simulink model "Model_2"  (R2020b)
settings: Solver=VariableStepAuto  StartTime=0.0  StopTime=10  RelTol=1e-3
values from neighbouring files (symbols this model uses):
  b1 = 350    [Variables.m]
  k1 = 80000    [Variables.m]
  k2 = 500000    [Variables.m]
  M1 = 2500    [Variables.m]
  M2 = 250    [Variables.m]
settings Model: SimulationMode=accelerator  Creator=samar  LastModifiedBy=samar

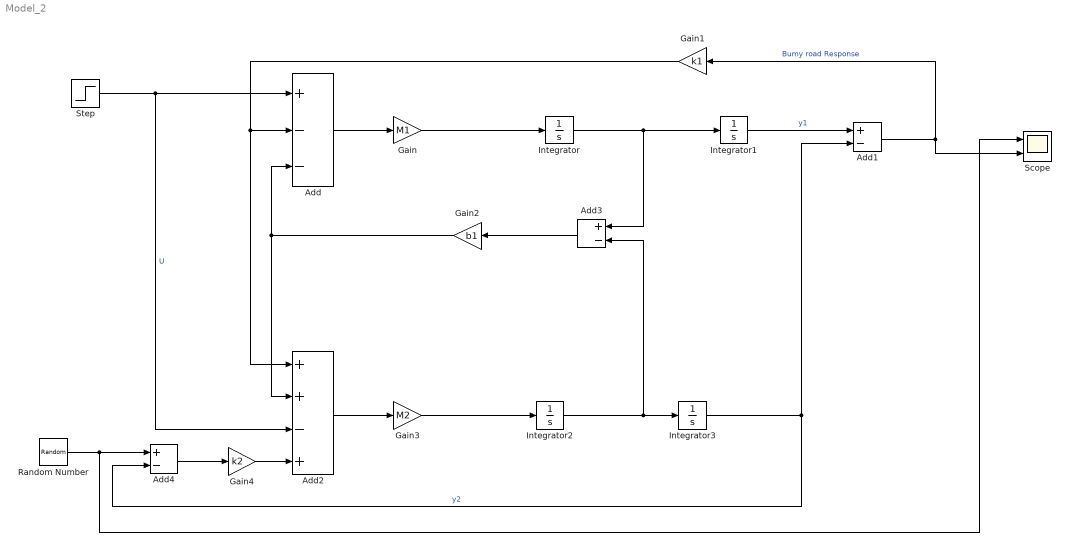
== system Model_2 ==
  Add : Sum  Inputs=+--
  Add1 : Sum  Inputs=+-
  Add2 : Sum  Inputs=++-+
  Add3 : Sum  Inputs=+-
  Add4 : Sum  Inputs=+-
  Gain : Gain  Gain=M1
  Gain1 : Gain  Gain=k1
  Gain2 : Gain  Gain=b1
  Gain3 : Gain  Gain=M2
  Gain4 : Gain  Gain=k2
  Integrator{,1..3} (4 alike) : Integrator
  Random Number : RandomNumber  SampleTime=0.1
  Scope : Scope  NumInputPorts=2
  Step : Step  SampleTime=0
  wires:
  Step/1 -> Add2/3, Add/1  "U"
  Add/1 -> Gain/1
  Integrator/1 -> Integrator1/1, Add3/1
  Gain/1 -> Integrator/1
  Integrator1/1 -> Add1/1  "y1"
  Add1/1 -> Gain1/1, Scope/2  "Bumy road Response"
  Gain1/1 -> Add2/1, Add/2
  Add3/1 -> Gain2/1
  Gain2/1 -> Add2/2, Add/3
  Add2/1 -> Gain3/1
  Gain3/1 -> Integrator2/1
  Integrator2/1 -> Add3/2, Integrator3/1
  Integrator3/1 -> Add4/2, Add1/2  "y2"
  Add4/1 -> Gain4/1
  Gain4/1 -> Add2/4
  Random Number/1 -> Scope/1, Add4/1
